simulink model "PVArrayGrid"  (R2024b)
settings: Solver=ode45  StartTime=0.0  StopTime=1.3  FixedStep=1  RelTol=1e-3
PreLoadFcn:
  | Ts_Power=1e-6;
  | Ts_Control=100e-6;
InitFcn:
  | Ts_Power=1e-6;
  | Ts_Control=100e-6;
undefined symbols (not defined in the file or in its folder): D1, Delta, DiscIntNeverNeededParam
libraries: spsSeriesRLCBranchLib x5, spsMeanLib x3, spsThreePhaseTransformerTwoWindingsLib x2, spsDistributedParametersLineLib x2, spsThreePhaseParallelRLCLoadLib x2, spsFourierLib x2, slpidlib x2, spsabctodq0Lib x2, spsVoltageMeasurementLib x2, spsThreePhaseSeriesRLCLoadLib x1, spsThreeLevelBridgeLib x1, spsThreePhaseSourceLib x1
(part 1 of 2)
settings Model: SimulationMode=accelerator  Creator=The MathWorks, Inc.  LastModifiedBy=shrot
settings SolverCC: AlgebraicLoopSolver=TrustRegion
settings DataIOCC: LimitDataPoints=on  SaveFormat=Array  SignalLogging=off  DSMLogging=off  ReturnWorkspaceOutputs=off
settings OptimizationCC: ExpressionDepthLimit=2147483647  EfficientMapNaN2IntZero=off  LifeSpan=inf
settings DebuggingCC: UnderspecifiedInitializationDetection=Classic  MergeDetectMultiDrivingBlocksExec=none  SolverPrmCheckMsg=warning  FcnCallInpInsideContextMsg=warning  UnconnectedInputMsg=warning  UnconnectedOutputMsg=warning  UnconnectedLineMsg=warning  StateNameClashWarn=warning  SubsystemReferenceDiagnosticForUnitTest=warning  SFUnexpectedBacktrackingDiag=warning  SFNoUnconditionalDefaultTransitionDiag=warning  SFExecutionAtInitializationDiag=none  ArithmeticOperatorsInVariantConditions=warning
settings HardwareCC: ProdBitPerPointer=32  ProdBitPerSizeT=32  ProdBitPerPtrDiffT=32  ProdLargestAtomicFloat=None  ProdIntDivRoundTo=Undefined  ProdEndianess=Unspecified  ProdWordSize=32  ProdHWDeviceType=32-bit Generic  TargetBitPerPointer=64  TargetBitPerSizeT=64  TargetBitPerPtrDiffT=64  TargetLongLongMode=on  TargetIntDivRoundTo=Zero  TargetEndianess=LittleEndian  TargetWordSize=64  TargetHWDeviceType=MATLAB Host  ProdEqTarget=off
settings ModelReferenceCC: EnableRefExpFcnMdlSchedulingChecks=on  PropagateSignalLabelsOutOfModel=off
settings SFSimCC: SimUseLocalCustomCode=off  CustomCodeUndefinedFunction=UseInterfaceOnly
settings RTWCC: GPUComputeCapability=3.5
settings CodeAppCC: MaxIdLength=128
settings GRTTargetCC: TargetLangStandard=C89/C90 (ANSI)  CombineOutputUpdateFcns=off  GRTInterface=on
settings ConfigComp: CovMetricSettings=dw  CovSaveCumulativeToWorkspaceVar=on  CovSaveSingleToWorkspaceVar=on  CovExternalEMLEnable=off  CovSFcnEnable=off
settings SimscapeCC: SimscapeNormalizeSystem=off

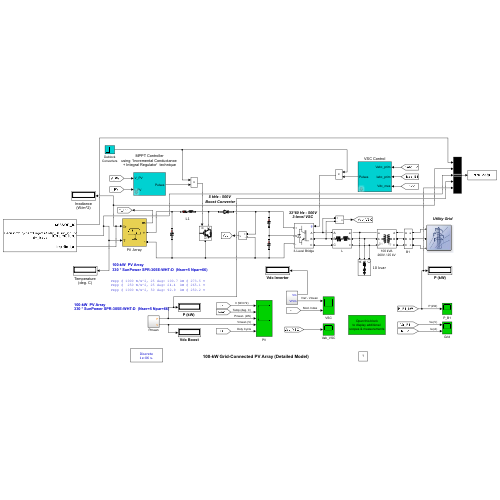
[thumbnail: Simulink's stored preview of the top-level diagram]
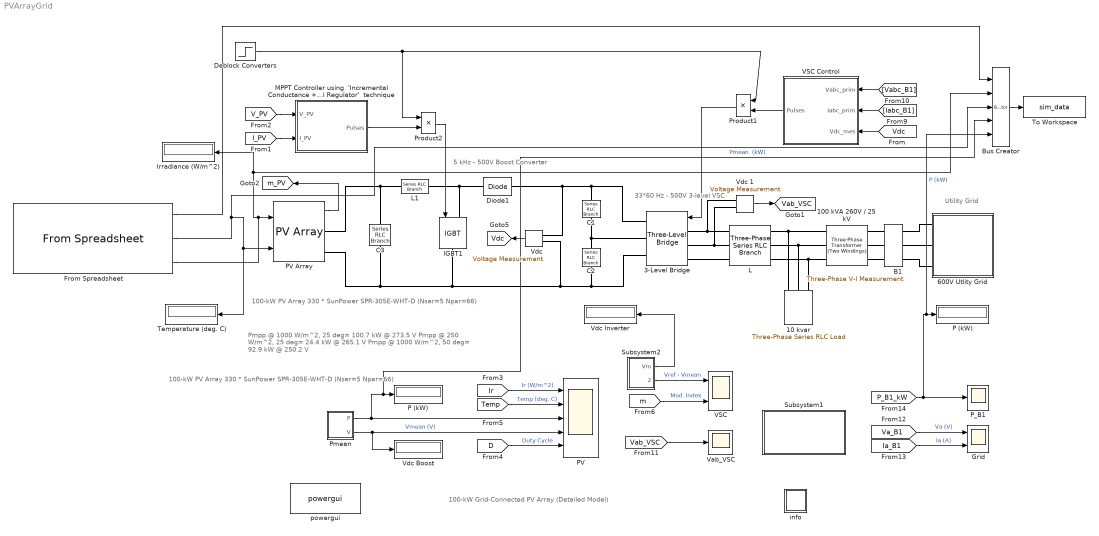
== system PVArrayGrid ==
  note: 5 kHz - 500V
      | Boost Converter
  note: 33*60 Hz - 500V
      | 3-level VSC
  note: 100-kW Grid-Connected PV Array (Detailed Model)
  note: Utility Grid
  note: Pmpp @ 1000 W/m^2, 25 deg= 100.7 kW @ 273.5 V
      | Pmpp @  250 W/m^2, 25 deg= 24.4  kW @ 265.1 V
      | Pmpp @ 1000 W/m^2, 50 deg= 92.9  kW @ 250.2 V
  note: 100-kW  PV Array
      | 330 * SunPower SPR-305E-WHT-D  (Nser=5 Npar=66)
  note: 100-kW  PV Array
      | 330 * SunPower SPR-305E-WHT-D  (Nser=5 Npar=66)
  10 kvar : spsThreePhaseSeriesRLCLoadLib/Three-Phase Series RLC Load  LConnTagsString=A|B|C  Configuration=Y (grounded)  NominalVoltage=240  Vabc=[1e3 1e3 1e3]  Vabcp=[1e3 1e3 1e3]  NominalFrequency=60  UnbalancedPower=off  ActivePower=10e3/100  InductivePower=0  CapacitivePower=10e3  Pabc=[10e3 9e3 11e3]  QLabc=[100 90 110]  QCabc=[100 90 110]  Pabcp=[10e3 9e3 11e3]  QLabcp=[100 90 110]  QCabcp=[100 90 110]  Measurements=None  LoadType=constant Z
  100 kVA 260V / 25 kV : spsThreePhaseTransformerTwoWindingsLib/Three-Phase Transformer (Two Windings)  Winding1Connection=Yg  Winding2Connection=Delta (D1)  CoreType=Three single-phase transformers  SetSaturation=off  Hysteresis=off  DataFile='hysteresis'  SetInitialFlux=off  Measurements=None  UNITS=pu  NominalPower=[100e3 , 60 ]  Winding1=[ 25e3 , 0.001 , 0.03 ]  Winding2=[ 260 , 0.001 , 0.03 ]  Rm=500  Lm=500  L0=0.5  Saturation=[ 0,0 ; 0.0024,1.2 ; 1.0,1.52 ]  InitialFluxes=[ 0.8 , -0.8 , 0.7 ]  BreakLoop=off  DiscreteSolver=Trapezoidal iterative  DataType=off  TransfoNumber=0
  3-Level Bridge : spsThreeLevelBridgeLib/Three-Level Bridge  Arms=3  SnubberResistance=1e6  SbubberCapacitance=inf  Device=IGBT / Diodes  Ron=0.2e-3  ForwardVoltages="[  0  0 ]"  Measurements=None
      settings: AttributesFormatString=\n
  600V Utlity Grid : Subsystem
      mask Display: image('$imagefile')
  B1 : spsThreePhaseVIMeasurementLib/Three-Phase V-I Measurement  VoltageMeasurement=phase-to-ground  SetLabelV=on  LabelV=Vabc_B1  Vpu=off  VpuLL=off  CurrentMeasurement=yes  SetLabelI=on  LabelI=Iabc_B1  Ipu=off  Pbase=100e6  Vbase=500e3  OutputType=Magnitude  PhasorSimulation=off  PSBequivalent=0
  Bus Creator : BusCreator  Inputs=5
  C1 : spsSeriesRLCBranchLib/Series RLC Branch  LConnTagsString=__new0  RConnTagsString=__new0  BranchType=C  Resistance=1.0  Inductance=1.0  SetiL0=off  InitialCurrent=0  Capacitance=12000e-06  Setx0=off  InitialVoltage=0  Measurements=None
  C2 : spsSeriesRLCBranchLib/Series RLC Branch  LConnTagsString=__new0  RConnTagsString=__new0  BranchType=C  Resistance=1.0  Inductance=1.0  SetiL0=off  InitialCurrent=0  Capacitance=12000e-06  Setx0=off  InitialVoltage=0  Measurements=None
  C3 : spsSeriesRLCBranchLib/Series RLC Branch  LConnTagsString=__new0  RConnTagsString=__new0  BranchType=C  Resistance=1.0  Inductance=1.0  SetiL0=off  InitialCurrent=0  Capacitance=100e-6  Setx0=off  InitialVoltage=0  Measurements=Branch voltage
  Deblock Converters : Step  Time=0.05  SampleTime=0
  Diode1 : spsDiodeLib/Diode  Ron=1e-4  Lon=0  Vf=0  IC=0  UseSnubber=off  Rs=inf  Cs=inf  Measurements=off
  From Spreadsheet : FromSpreadsheet  FileName=C:\Users\shrot\PycharmProjects\Solar_DT\sim_input.csv  SheetName=sim_input  TreatFirstColumnAs=Data  SampleTime=4
  Grid : Scope  NumInputPorts=2
  IGBT1 : spsIGBTLib/IGBT  Ron=0.001  Lon=0  Vf=0  Tf=0  Tt=0  IC=0  Rs=1e5  Cs=inf  Measurements=off
  Irradiance (W/m^2) : Display
      settings: Format=bank  Decimation=1000
  L : spsThreePhaseSeriesRLCBranchLib/Three-Phase Series RLC Branch  LConnTagsString=A|B|C  RConnTagsString=A|B|C  BranchType=RL  Resistance=500e-6*377/50/2  Inductance=500e-6/2  Capacitance=inf  Measurements=None
  L1 : spsSeriesRLCBranchLib/Series RLC Branch  LConnTagsString=__new0  RConnTagsString=__new0  BranchType=RL  Resistance=0.005  Inductance=5e-3  SetiL0=off  InitialCurrent=0  Capacitance=1e-6  Setx0=off  InitialVoltage=0  Measurements=None
  "MPPT Controller using  'Incremental Conductance + Integral Regulator'  technique " : Subsystem  mask(Boost Control - MPPT){fc=5000, T_MPPT=200e-6, Dinit=0.5}
      mask prompts: fc "PWM switching frequency (Hz)"; T_MPPT "Time window used by MPPT control (s)"; Dinit "Initial value of duty cycle"
  P (kW) : Display
      settings: Format=bank  Decimation=2000
  "P (kW) " : Display
      settings: Format=bank  Decimation=2000
  PV : Scope  NumInputPorts=5
  PV Array : spsPVArrayLib/PV Array  Npar=66  Nser=5  PlotType=array @ 1000 W/m2 & specified temperatures  S_vec="[ 1000  250 ]"  Temp_C_vec="[0 25 50  ]"  ModuleName=SunPower SPR-305E-WHT-D  PlotWhenSelected=off  Pm=305.226  Ncell=96  Voc=64.2  Isc=5.96  Vm=54.7  Im=5.58  beta_Voc_pc=-0.2727  alpha_Isc_pc=0.061745  beta_Voc=-0.17507  alpha_Isc=0.00368  IL=5.9657  I0=6.3076e-12  nI=0.94489  Rsh=393.2054  Rs=0.37428  RobustModel=off  RobustCellTemperature=25  BAL=on  Tc=1e-6  Tfilter=5e-5
  P_B1 : Scope
  Pmean : Subsystem
  Product1 : Product  RndMeth=Zero
  Product2 : Product  RndMeth=Zero
  Subsystem1 : Subsystem
      mask Display: disp('Open this block\nto display additional \nscopes & measurements')
  Subsystem2 : Subsystem
  Temperature (deg. C) : Display
      settings: Format=bank  Decimation=1000
  To Workspace : ToWorkspace  VariableName=sim_data  SampleTime=-1
      settings: MaxDataPoints=1
  VSC : Scope  NumInputPorts=2
  VSC Control : Subsystem  mask(VSC Main Controller){nom=[ 100e3  60 ], Vnom=[ 25e3 260 ], Vnom_dc=500, RLxfo=[0.002  0.06 ], RLchoke=[2e-3  250e-6  ], K_VDCreg=[7  800], K_Ireg=[0.3 20], Ts=Ts_Control}
      mask prompts: nom "Nominal power and frequency [ Pnom(VA)  Fnom(Hz) ]:"; Vnom "Nominal primary and secondary voltages (Vrms LL) [ Vnom_prim   Vnom_sec ]:"; Vnom_dc "Nominal DC bus voltage (V):"; RLxfo "Total transformer leakage impedance (pu/Pnom) [ Rxfo  Lxf ]"; RLchoke "Choke impedance [ R(ohm) L(H) ]"; K_VDCreg "VDC regultator gains [ Kp  Ki ]:"; K_Ireg "Current regulator gains [ Kp  Ki ]:"; Ts "Sample time"
      mask init:
      | Pnom=nom(1);
      | Fnom=nom(2);
      | Vnom_prim=Vnom(1);
      | Vnom_sec=Vnom(2);
      | Zbase=Vnom_sec^2/Pnom;
      | Rtot_pu=RLxfo(1) + RLchoke(1)/Zbase;
      | Ltot_pu=RLxfo(2) + RLchoke(2)/(Zbase/(2*pi*Fnom));
      | Kp_VDCreg=K_VDCreg(1);
      | Ki_VDCreg=K_VDCreg(2);
      | Kp_Ireg=K_Ireg(1);
      | Ki_Ireg=K_Ireg(2);
      | Vdc_ref=Vnom_dc;
      | % Used to determine initial value of Boost Control (MPPT)
      | assignin('base','Vdc_ref_Inv',Vdc_ref);
  Vab_VSC : Scope
  "Vdc " : spsVoltageMeasurementLib/Voltage Measurement  Tag=PoWeRsYsTeMmEaSuReMeNt  PhasorSimulation=off  OutputType=Magnitude  PSBequivalent=0
  Vdc 1 : spsVoltageMeasurementLib/Voltage Measurement  Tag=PoWeRsYsTeMmEaSuReMeNt  PhasorSimulation=off  OutputType=Magnitude  PSBequivalent=0
  Vdc Boost : Display
      settings: Format=bank  Decimation=2000
  Vdc Inverter : Display
      settings: Format=bank  Decimation=2000
  info : Subsystem
      settings: OpenFcn="showExample(\"simscapeelectricalsps/PVArrayGridExample\")"
      mask Display: disp('?')
  powergui : spspowerguiLib/powergui  Priority=1  SimulationMode=Discrete  SampleTime=Ts_Power  frequency=60  Iterations=50  frequencyindice=0  Pbase=100e6  ErrMax=1e-4  UnitsV=kV  UnitsW=MW  buscounter=0  FunctionMessages=off  echomessages=off  EnableUseOfTLC=off  CurrentSourceSwitches=off  DisableSnubberDevices=off  DisableRonSwitches=off  DisableVfSwitches=off  DisplayEquations=off  AutomaticDiscreteSolvers=off  SolverType=Tustin/Backward Euler (TBE)  Interpol=off  ExternalGateDelay=off  methode=off  Ts=0  x0status=blocks  SPID=off  SwTol=0  HookPort=off  NonlinearTolerance=1e-8  nMaxIteration=10  ContinueOnMaxIteration=off  RestoreLinks=warning  ResistiveCurrentMeasurement=off  Frange=[0:2:500]  Ylog=off  Xlog=on  ShowGrid=off  save=off  variable=ZData  structure=0  ZoomFFT=on  StartTime=0.0  cycles=1  DisplayStyle=1  fundamental=60  FreqAxis=off  MaxFrequency=1000  frequencyindicesteady=1  RmsSteady=1  display=off
  tag scope: Vab_VSC=global, Vdc=global, m_PV=global
  wires:
  "Vdc "/1 -> [Vdc]
  Product2/1 -> IGBT1/1
  "MPPT Controller using  'Incremental Conductance + Integral Regulator'  technique "/1(Pulses) -> Product2/2
  Deblock Converters/1 -> Product1/1, Product2/1
  [Vabc_B1] -> VSC Control/1(Vabc_prim)
  [Iabc_B1] -> VSC Control/2(Iabc_prim)
  [Vdc] -> VSC Control/3(Vdc_mes)
  VSC Control/1(Pulses) -> Product1/2
  Product1/1 -> 3-Level Bridge/1
  [I_PV] -> "MPPT Controller using  'Incremental Conductance + Integral Regulator'  technique "/2(I_PV)
  [V_PV] -> "MPPT Controller using  'Incremental Conductance + Integral Regulator'  technique "/1(V_PV)
  Pmean/1(P) -> Bus Creator/4, "P (kW) "/1, PV/3  "Pmean  (kW)"
  [m] -> VSC/2  "Mod. Index"
  Vdc 1/1 -> [Vab_VSC]
  [Vab_VSC] -> Vab_VSC/1
  [Ia_B1] -> Grid/2  "Ia (A)"
  [Va_B1] -> Grid/1  "Va (V)"
  [P_B1_kW] -> P_B1/1, Bus Creator/5, P (kW)/1  "P (kW)"
  Pmean/2(V) -> Vdc Boost/1, PV/4  "Vmean (V)"
  Subsystem2/2(VrVm) -> VSC/1  "Vref - Vmean"
  Subsystem2/1(Vm) -> Vdc Inverter/1
  PV Array/1 -> [m_PV]
  From Spreadsheet/2 -> Bus Creator/3, Temperature (deg. C)/1, PV Array/2
  [D] -> PV/5  "Duty Cycle"
  [Temp] -> PV/2  "Temp (deg. C)"
  [Ir] -> PV/1  "Ir (W/m^2)"
  Bus Creator/1 -> To Workspace/1
  From Spreadsheet/3 -> PV Array/1, Bus Creator/2, Irradiance (W/m^2)/1
  From Spreadsheet/1 -> Bus Creator/1
  connections:
  3-Level Bridge/RConn1 -- Diode1/RConn1 -- "Vdc "/LConn1 -- C1/LConn1
  L1/RConn1 -- Diode1/LConn1 -- IGBT1/LConn1
  3-Level Bridge/RConn3 -- C2/RConn1 -- "Vdc "/LConn2 -- IGBT1/RConn1 -- PV Array/RConn2 -- C3/RConn1
  3-Level Bridge/LConn1 -- L/LConn1 -- Vdc 1/LConn1
  3-Level Bridge/LConn2 -- L/LConn2 -- Vdc 1/LConn2
  3-Level Bridge/LConn3 -- L/LConn3
  L/RConn1 -- 100 kVA 260V / 25 kV/RConn1 -- 10 kvar/LConn1
  L/RConn2 -- 100 kVA 260V / 25 kV/RConn2 -- 10 kvar/LConn2
  L/RConn3 -- 100 kVA 260V / 25 kV/RConn3 -- 10 kvar/LConn3
  B1/LConn1 -- 100 kVA 260V / 25 kV/LConn1
  B1/LConn2 -- 100 kVA 260V / 25 kV/LConn2
  B1/LConn3 -- 100 kVA 260V / 25 kV/LConn3
  C2/LConn1 -- C1/RConn1 -- 3-Level Bridge/RConn2
  C3/LConn1 -- PV Array/RConn1 -- L1/LConn1
  B1/RConn2 -- 600V Utlity Grid/LConn2
  B1/RConn1 -- 600V Utlity Grid/LConn1
  B1/RConn3 -- 600V Utlity Grid/LConn3

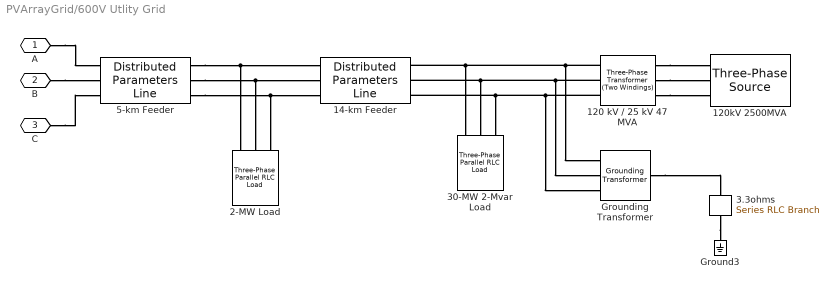
== system PVArrayGrid/600V Utlity Grid ==
  120 kV / 25 kV 47 MVA : spsThreePhaseTransformerTwoWindingsLib/Three-Phase Transformer (Two Windings)  Winding1Connection=Yg  Winding2Connection=Delta (D1)  CoreType=Three single-phase transformers  SetSaturation=off  Hysteresis=off  DataFile='basic_model'  SetInitialFlux=off  Measurements=None  UNITS=pu  NominalPower=[47e6 60 ]  Winding1="[ 120e3  0.08/30   0.08 ]"  Winding2="[ 25e3  0.08/30  0.08]"  Rm=500  Lm=500  L0=0.5  Saturation="[ 0,0  ;  0.005,1.2  ;  1.0,1.4 ]"  InitialFluxes=[ 0.8 , -0.8 , 0.7 ]  BreakLoop=off  DiscreteSolver=Trapezoidal iterative  DataType=off  TransfoNumber=0
  120kV 2500MVA : spsThreePhaseSourceLib/Three-Phase Source  InternalConnection=Yg  VoltagePhases=off  Voltage=120e3  PhaseAngle=0  Voltage_phases=[25e3 25e3 25e3]/sqrt(3)  PhaseAngles_phases=[0 -120 +120]  Frequency=60  NonIdealSource=on  SpecifyImpedance=on  Resistance=0.8929  Inductance=16.58e-3  ShortCircuitLevel=2500e6  BaseVoltage=120e3  XRratio=7  BusType=swing  Pref=0  Qref=0  Prefabc=[10e3, 10e3, 10e3]  Qrefabc=[0, 0, 0]  Qmin=-inf  Qmax=inf
  14-km Feeder : spsDistributedParametersLineLib/Distributed Parameters Line  Phases=3  Length=14  Frequency=60  Resistance=[0.1153 0.413]  Inductance=[1.05e-3 3.32e-3]  Capacitance=[11.33e-009 5.01e-009]  x1=[-5.8e-05 1.09765853041463e-09 0 0;-5.7e-05 1.09777450341744e-09 0 0;-5.6e-05 1.09789032040201e-09 0 0;-5.5e-05 1.09800598135188e-09 0 0;-5.4e-05 1.09812148625062e-09 0 0;-5.3e-05 1.0982368350818e-09 0 0;-5.2e-05 1.09835202782904e-09 0 0;-5.1e-05 1.09846706447595e-09 0 0;-5e-05 1.0985819450062e-09 0 0;-4.9e-05 1.09869666940346e-09 -3790.73535189818 -24061.4134200269;-4.8e-05 1.09881123765141e-09 -3781.66414358279 -24062.8407837213;-4.7e-05 1.09892564973379e-09 -3772.59239780858 -24064.2647275494;-4.6e-05 1.09903990563432e-09 -3763.52011586486 -24065.6852513088;-4.5e-05 1.09915400533677e-09 -3754.447299041 -24067.1023547976;-4.4e-05 1.09926794882492e-09 -3745.37394862644 -24068.5160378144;-4.3e-05 1.09938173608258e-09 -3736.30006591072 -24069.9263001584;-4.2e-05 1.09949536709358e-09 -3727.22565218343 -24071.333141629;-4.1e-05 1.09960884184177e-09 -3718.15070873426 -24072.7365620263;-4e-05 1.09972216031101e-09 -3709.07523685295 -24074.1365611509;-3.9e-05 1.09983532248522e-09 -3699.99923782933 -24075.5331388038;-3.8e-05 1.09994832834829e-09 -3690.9227129533 -24076.9262947866;-3.7e-05 1.10006117788418e-09 -3681.84566351484 -24078.3160289011;-3.6e-05 1.10017387107684e-09 -3672.768090804 -24079.70234095;-3.5e-05 1.10028640791025e-09 -3663.6899961109 -24081.0852307361;-3.4e-05 1.10039878836843e-09 -3654.61138072575 -24082.464698063;-3.3e-05 1.10051101243541e-09 -3645.53224593882 -24083.8407427345;-3.2e-05 1.10062308009522e-09 -3636.45259304045 -24085.2133645552;-3.1e-05 1.10073499133195e-09 -3627.37242332107 -24086.5825633299;-3e-05 1.10084674612968e-09 -3618.29173807118 -24087.9483388641;-2.9e-05 1.10095834447255e-09 -3609.21053858133 -24089.3106909636;-2.8e-05 1.10106978634468e-09 -3600.12882614218 -24090.6696194348;-2.7e-05 1.10118107173024e-09 -3591.04660204443 -24092.0251240846;-2.6e-05 1.10129220061341e-09 -3581.96386757887 -24093.3772047204;-2.5e-05 1.10140317297839e-09 -3572.88062403636 -24094.7258611499;-2.4e-05 1.10151398880943e-09 -3563.79687270783 -24096.0710931815;-2.3e-05 1.10162464809076e-09 -3554.71261488429 -24097.412900624;-2.2e-05 1.10173515080665e-09 -3545.62785185682 -24098.7512832868;-2.1e-05 1.10184549694142e-09 -3536.54258491655 -24100.0862409795;-2e-05 1.10195568647936e-09 -3527.4568153547 -24101.4177735126;-1.9e-05 1.10206571940483e-09 -3518.37054446258 -24102.7458806966;-1.8e-05 1.10217559570218e-09 -3509.28377353153 -24104.0705623429;-1.7e-05 1.1022853153558e-09 -3500.196503853 -24105.3918182633;-1.6e-05 1.10239487835009e-09 -3491.10873671849 -24106.7096482699;-1.5e-05 1.10250428466948e-09 -3482.02047341956 -24108.0240521754;-1.4e-05 1.10261353429843e-09 -3472.93171524788 -24109.335029793;-1.3e-05 1.1027226272214e-09 -3463.84246349514 -24110.6425809365;-1.2e-05 1.1028315634229e-09 -3454.75271945314 -24111.9467054199;-1.1e-05 1.10294034288744e-09 -3445.66248441373 -24113.247403058;-1e-05 1.10304896559955e-09 -3436.57175966884 -24114.5446736659;-9e-06 1.10315743154381e-09 -3427.48054651046 -24115.8385170591;-8e-06 1.10326574070479e-09 -3418.38884623065 -24117.1289330539;-7e-06 1.10337389306711e-09 -3409.29666012156 -24118.4159214668;-6e-06 1.10348188861539e-09 -3400.20398947537 -24119.6994821149;-5e-06 1.10358972733429e-09 -3391.11083558437 -24120.9796148158;-4e-06 1.10369740920847e-09 -3382.01719974089 -24122.2563193876;-3e-06 1.10380493422264e-09 -3372.92308323734 -24123.5295956488;-2e-06 1.10391230236151e-09 -3363.8284873662 -24124.7994434184;-1e-06 1.10401951360982e-09 -3354.73341342002 -24126.0658625161]  x2=[-5.8e-05 1.13481958980174e-09 0 0;-5.7e-05 1.13493792425514e-09 0 0;-5.6e-05 1.13505609740854e-09 0 0;-5.5e-05 1.13517410924515e-09 0 0;-5.4e-05 1.13529195974821e-09 0 0;-5.3e-05 1.13540964890097e-09 0 0;-5.2e-05 1.13552717668669e-09 0 0;-5.1e-05 1.13564454308867e-09 0 0;-5e-05 1.13576174809024e-09 0 0;-4.9e-05 1.13587879167473e-09 -3379.39242591167 -24244.051273217;-4.8e-05 1.13599567382552e-09 -3370.25239397986 -24245.3235513069;-4.7e-05 1.13611239452599e-09 -3361.11188306003 -24246.5923835956;-4.6e-05 1.13622895375954e-09 -3351.97089445124 -24247.8577699028;-4.5e-05 1.13634535150963e-09 -3342.82942945264 -24249.1197100486;-4.4e-05 1.13646158775969e-09 -3333.68748936342 -24250.3782038537;-4.3e-05 1.13657766249322e-09 -3324.54507548286 -24251.6332511393;-4.2e-05 1.13669357569372e-09 -3315.4021891103 -24252.8848517269;-4.1e-05 1.13680932734471e-09 -3306.25883154515 -24254.1330054387;-4e-05 1.13692491742974e-09 -3297.11500408689 -24255.3777120973;-3.9e-05 1.13704034593239e-09 -3287.97070803506 -24256.6189715258;-3.8e-05 1.13715561283624e-09 -3278.82594468926 -24257.8567835478;-3.7e-05 1.13727071812492e-09 -3269.68071534916 -24259.0911479873;-3.6e-05 1.13738566178207e-09 -3260.53502131452 -24260.322064669;-3.5e-05 1.13750044379135e-09 -3251.38886388514 -24261.5495334178;-3.4e-05 1.13761506413645e-09 -3242.24224436089 -24262.7735540594;-3.3e-05 1.13772952280108e-09 -3233.09516404171 -24263.9941264198;-3.2e-05 1.13784381976897e-09 -3223.9476242276 -24265.2112503254;-3.1e-05 1.13795795502387e-09 -3214.79962621864 -24266.4249256034;-3e-05 1.13807192854958e-09 -3205.65117131495 -24267.6351520813;-2.9e-05 1.13818574032988e-09 -3196.50226081674 -24268.8419295869;-2.8e-05 1.1382993903486e-09 -3187.35289602427 -24270.0452579489;-2.7e-05 1.1384128785896e-09 -3178.20307823788 -24271.2451369962;-2.6e-05 1.13852620503673e-09 -3169.05280875794 -24272.4415665583;-2.5e-05 1.1386393696739e-09 -3159.90208888493 -24273.6345464651;-2.4e-05 1.13875237248503e-09 -3150.75091991935 -24274.8240765471;-2.3e-05 1.13886521345404e-09 -3141.59930316181 -24276.0101566352;-2.2e-05 1.13897789256491e-09 -3132.44723991294 -24277.1927865609;-2.1e-05 1.13909040980162e-09 -3123.29473147346 -24278.3719661561;-2e-05 1.13920276514818e-09 -3114.14177914414 -24279.5476952531;-1.9e-05 1.13931495858862e-09 -3104.98838422583 -24280.719973685;-1.8e-05 1.13942699010699e-09 -3095.83454801942 -24281.888801285;-1.7e-05 1.13953885968738e-09 -3086.68027182588 -24283.0541778872;-1.6e-05 1.13965056731389e-09 -3077.52555694623 -24284.2161033257;-1.5e-05 1.13976211297063e-09 -3068.37040468157 -24285.3745774356;-1.4e-05 1.13987349664176e-09 -3059.21481633304 -24286.5296000522;-1.3e-05 1.13998471831144e-09 -3050.05879320186 -24287.6811710113;-1.2e-05 1.14009577796387e-09 -3040.90233658931 -24288.8292901492;-1.1e-05 1.14020667558326e-09 -3031.74544779671 -24289.9739573028;-1e-05 1.14031741115386e-09 -3022.58812812548 -24291.1151723093;-9e-06 1.14042798465992e-09 -3013.43037887706 -24292.2529350067;-8e-06 1.14053839608573e-09 -3004.27220135299 -24293.3872452332;-7e-06 1.1406486454156e-09 -2995.11359685483 -24294.5181028276;-6e-06 1.14075873263386e-09 -2985.95456668423 -24295.6455076291;-5e-06 1.14086865772486e-09 -2976.7951121429 -24296.7694594776;-4e-06 1.14097842067298e-09 -2967.6352345326 -24297.8899582133;-3e-06 1.14108802146262e-09 -2958.47493515514 -24299.0070036769;-2e-06 1.14119746007821e-09 -2949.31421531242 -24300.1205957098;-1e-06 1.14130673650419e-09 -2940.15307630637 -24301.2307341535]  x3=[-5.8e-05 1.57399423716255e-12 0 0;-5.7e-05 1.57518382731474e-12 0 0;-5.6e-05 1.57637319359817e-12 0 0;-5.5e-05 1.57756233584382e-12 0 0;-5.4e-05 1.57875125388268e-12 0 0;-5.3e-05 1.57993994754577e-12 0 0;-5.2e-05 1.58112841666416e-12 0 0;-5.1e-05 1.58231666106895e-12 0 0;-5e-05 1.58350468059125e-12 0 0;-4.9e-05 1.58469247506221e-12 -23.5442847382529 -155.681477773836;-4.8e-05 1.58588004431304e-12 -23.4855925321342 -155.690342696957;-4.7e-05 1.58706738817494e-12 -23.4268969881891 -155.699185493008;-4.6e-05 1.58825450647917e-12 -23.3681981147594 -155.708006160732;-4.5e-05 1.58944139905702e-12 -23.3094959201876 -155.716804698876;-4.4e-05 1.5906280657398e-12 -23.2507904128166 -155.72558110619;-4.3e-05 1.59181450635885e-12 -23.1920816009898 -155.734335381425;-4.2e-05 1.59300072074557e-12 -23.1333694930509 -155.743067523339;-4.1e-05 1.59418670873135e-12 -23.0746540973444 -155.751777530689;-4e-05 1.59537247014765e-12 -23.0159354222148 -155.760465402238;-3.9e-05 1.59655800482594e-12 -22.9572134760076 -155.769131136751;-3.8e-05 1.59774331259774e-12 -22.8984882670684 -155.777774732996;-3.7e-05 1.59892839329458e-12 -22.8397598037432 -155.786396189746;-3.6e-05 1.60011324674803e-12 -22.7810280943789 -155.794995505775;-3.5e-05 1.60129787278971e-12 -22.7222931473224 -155.80357267986;-3.4e-05 1.60248227125124e-12 -22.6635549709213 -155.812127710783;-3.3e-05 1.60366644196431e-12 -22.6048135735236 -155.820660597327;-3.2e-05 1.60485038476061e-12 -22.5460689634778 -155.829171338281;-3.1e-05 1.60603409947188e-12 -22.4873211491327 -155.837659932434;-3e-05 1.60721758592989e-12 -22.4285701388378 -155.84612637858;-2.9e-05 1.60840084396644e-12 -22.3698159409429 -155.854570675516;-2.8e-05 1.60958387341335e-12 -22.3110585637983 -155.862992822042;-2.7e-05 1.61076667410251e-12 -22.2522980157547 -155.871392816961;-2.6e-05 1.61194924586579e-12 -22.1935343051632 -155.879770659078;-2.5e-05 1.61313158853514e-12 -22.1347674403756 -155.888126347204;-2.4e-05 1.61431370194251e-12 -22.0759974297439 -155.89645988015;-2.3e-05 1.6154955859199e-12 -22.0172242816206 -155.904771256732;-2.2e-05 1.61667724029935e-12 -21.9584480043588 -155.91306047577;-2.1e-05 1.6178586649129e-12 -21.8996686063117 -155.921327536085;-2e-05 1.61903985959265e-12 -21.8408860958334 -155.929572436501;-1.9e-05 1.62022082417074e-12 -21.782100481278 -155.937795175848;-1.8e-05 1.62140155847931e-12 -21.7233117710004 -155.945995752956;-1.7e-05 1.62258206235056e-12 -21.6645199733557 -155.954174166661;-1.6e-05 1.62376233561671e-12 -21.6057250966996 -155.9623304158;-1.5e-05 1.62494237811002e-12 -21.5469271493881 -155.970464499213;-1.4e-05 1.62612218966278e-12 -21.4881261397777 -155.978576415744;-1.3e-05 1.62730177010731e-12 -21.4293220762254 -155.986666164242;-1.2e-05 1.62848111927597e-12 -21.3705149670885 -155.994733743555;-1.1e-05 1.62966023700114e-12 -21.3117048207248 -156.002779152538;-1e-05 1.63083912311525e-12 -21.2528916454926 -156.010802390047;-9e-06 1.63201777745075e-12 -21.1940754497505 -156.018803454941;-8e-06 1.63319619984013e-12 -21.1352562418576 -156.026782346084;-7e-06 1.63437439011591e-12 -21.0764340301734 -156.034739062341;-6e-06 1.63555234811063e-12 -21.017608823058 -156.042673602583;-5e-06 1.63673007365689e-12 -20.9587806288716 -156.05058596568;-4e-06 1.6379075665873e-12 -20.899949455975 -156.058476150509;-3e-06 1.63908482673453e-12 -20.8411153127295 -156.066344155948;-2e-06 1.64026185393124e-12 -20.7822782074968 -156.074189980879;-1e-06 1.64143864801016e-12 -20.7234381486388 -156.082013624187]  x4=[-5.8e-05 1.05853260132924e-12 0 0;-5.7e-05 1.0580479194887e-12 0 0;-5.6e-05 1.05756308727595e-12 0 0;-5.5e-05 1.0570781047599e-12 0 0;-5.4e-05 1.05659297200948e-12 0 0;-5.3e-05 1.05610768909363e-12 0 0;-5.2e-05 1.05562225608133e-12 0 0;-5.1e-05 1.05513667304156e-12 0 0;-5e-05 1.05465094004334e-12 0 0;-4.9e-05 1.0541650571557e-12 -1.35581366009422 -2.15298522698177;-4.8e-05 1.05367902444769e-12 -1.35500190745908 -2.15349620368416;-4.7e-05 1.0531928419884e-12 -1.35418996224795 -2.15400687432671;-4.6e-05 1.05270650984692e-12 -1.35337782457623 -2.15451723883685;-4.5e-05 1.05222002809236e-12 -1.35256549455934 -2.15502729714204;-4.4e-05 1.05173339679387e-12 -1.35175297231272 -2.15553704916979;-4.3e-05 1.05124661602062e-12 -1.35094025795186 -2.15604649484765;-4.2e-05 1.05075968584177e-12 -1.35012735159227 -2.15655563410322;-4.1e-05 1.05027260632654e-12 -1.34931425334946 -2.15706446686414;-4e-05 1.04978537754414e-12 -1.34850096333901 -2.1575729930581;-3.9e-05 1.04929799956384e-12 -1.3476874816765 -2.15808121261281;-3.8e-05 1.04881047245488e-12 -1.34687380847754 -2.15858912545605;-3.7e-05 1.04832279628657e-12 -1.34605994385778 -2.15909673151564;-3.6e-05 1.04783497112821e-12 -1.34524588793287 -2.15960403071944;-3.5e-05 1.04734699704913e-12 -1.34443164081853 -2.16011102299533;-3.4e-05 1.04685887411869e-12 -1.34361720263047 -2.16061770827128;-3.3e-05 1.04637060240625e-12 -1.34280257348443 -2.16112408647527;-3.2e-05 1.04588218198121e-12 -1.34198775349621 -2.16163015753532;-3.1e-05 1.04539361291299e-12 -1.3411727427816 -2.16213592137952;-3e-05 1.04490489527103e-12 -1.34035754145642 -2.16264137793599;-2.9e-05 1.04441602912477e-12 -1.33954214963655 -2.16314652713289;-2.8e-05 1.04392701454371e-12 -1.33872656743787 -2.16365136889843;-2.7e-05 1.04343785159734e-12 -1.33791079497629 -2.16415590316085;-2.6e-05 1.04294854035517e-12 -1.33709483236774 -2.16466012984845;-2.5e-05 1.04245908088676e-12 -1.3362786797282 -2.16516404888958;-2.4e-05 1.04196947326167e-12 -1.33546233717366 -2.1656676602126;-2.3e-05 1.04147971754947e-12 -1.33464580482013 -2.16617096374595;-2.2e-05 1.04098981381978e-12 -1.33382908278368 -2.1666739594181;-2.1e-05 1.04049976214223e-12 -1.33301217118036 -2.16717664715756;-2e-05 1.04000956258645e-12 -1.33219507012628 -2.16767902689289;-1.9e-05 1.03951921522212e-12 -1.33137777973758 -2.16818109855268;-1.8e-05 1.03902872011892e-12 -1.3305603001304 -2.16868286206559;-1.7e-05 1.03853807734658e-12 -1.32974263142093 -2.1691843173603;-1.6e-05 1.03804728697481e-12 -1.32892477372537 -2.16968546436553;-1.5e-05 1.03755634907337e-12 -1.32810672715997 -2.17018630301008;-1.4e-05 1.03706526371203e-12 -1.32728849184098 -2.17068683322275;-1.3e-05 1.03657403096059e-12 -1.3264700678847 -2.17118705493242;-1.2e-05 1.03608265088887e-12 -1.32565145540744 -2.17168696806798;-1.1e-05 1.03559112356669e-12 -1.32483265452554 -2.17218657255839;-1e-05 1.03509944906392e-12 -1.32401366535538 -2.17268586833265;-9e-06 1.03460762745043e-12 -1.32319448801334 -2.17318485531979;-8e-06 1.03411565879613e-12 -1.32237512261586 -2.1736835334489;-7e-06 1.03362354317093e-12 -1.32155556927938 -2.17418190264909;-6e-06 1.03313128064477e-12 -1.32073582812039 -2.17467996284956;-5e-06 1.03263887128761e-12 -1.31991589925538 -2.1751777139795;-4e-06 1.03214631516945e-12 -1.31909578280088 -2.17567515596818;-3e-06 1.03165361236027e-12 -1.31827547887345 -2.17617228874489;-2e-06 1.0311607629301e-12 -1.31745498758968 -2.176669112239;-1e-06 1.030667766949e-12 -1.31663430906618 -2.17716562637988]  x5=5.70973484498186e-05  V1=[0 0 0 2.868e-09 2.436e+04 2.436e+04;0 0 0 377 377 377;1.571 1.571 1.571 -0.5389 -0.156 -1.727]  V2=[0 0 0 2.996e-09 2.448e+04 2.448e+04;0 0 0 377 377 377;1.571 1.571 1.571 -0.5232 -0.1382 -1.709]  I1=[0 0 0 1.022e-11 157.5 157.5;0 0 0 377 377 377;1.571 1.571 1.571 -1.198 -0.1498 -1.721]  I2=[0 0 0 6.231e-12 2.544 2.544;0 0 0 377 377 377;1.571 1.571 1.571 1.184 -0.5617 -2.133]  nHarmo=2  Measurements=None  Decoupling=off  VsMag0=0  VrMag0=0  VsAngle0=0  VrAngle0=0  IsMag0=0  IrMag0=0  IsAngle0=0  IrAngle0=0
  2-MW Load : spsThreePhaseParallelRLCLoadLib/Three-Phase Parallel RLC Load  LConnTagsString=A|B|C  Configuration=Y (grounded)  NominalVoltage=25e3  Vabc=[1e3 1e3 1e3]  Vabcp=[1e3 1e3 1e3]  NominalFrequency=60  UnbalancedPower=off  ActivePower=2e6  InductivePower=0  CapacitivePower=0  Pabc=[10e3 9e3 11e3]  QLabc=[100 90 110]  QCabc=[100 90 110]  Pabcp=[10e3 9e3 11e3]  QLabcp=[100 90 110]  QCabcp=[100 90 110]  Measurements=None  LoadType=constant Z
  "3.3ohms " : spsSeriesRLCBranchLib/Series RLC Branch  LConnTagsString=__new0  RConnTagsString=__new0  BranchType=R  Resistance=3.3  Inductance=[]  SetiL0=off  InitialCurrent=0  Capacitance=[]  Setx0=off  InitialVoltage=0  Measurements=None
  30-MW 2-Mvar Load : spsThreePhaseParallelRLCLoadLib/Three-Phase Parallel RLC Load  LConnTagsString=A|B|C  Configuration=Y (grounded)  NominalVoltage=25e3  Vabc=[1e3 1e3 1e3]  Vabcp=[1e3 1e3 1e3]  NominalFrequency=60  UnbalancedPower=off  ActivePower=30e6  InductivePower=2e6  CapacitivePower=0  Pabc=[10e3 9e3 11e3]  QLabc=[100 90 110]  QCabc=[100 90 110]  Pabcp=[10e3 9e3 11e3]  QLabcp=[100 90 110]  QCabcp=[100 90 110]  Measurements=None  LoadType=constant Z
  5-km Feeder : spsDistributedParametersLineLib/Distributed Parameters Line  Phases=3  Length=5  Frequency=60  Resistance=[0.1153 0.413]  Inductance=[1.05e-3 3.32e-3]  Capacitance=[11.33e-009 5.01e-009]  x1=[-2.1e-05 1.08380017743144e-09 -3537.17773129479 -24101.4118174708;-2e-05 1.08390345674986e-09 -3528.09146195726 -24102.7435893542;-1.9e-05 1.08400658202142e-09 -3519.00469119925 -24104.0719357001;-1.8e-05 1.08410955323147e-09 -3509.9174203122 -24105.3968563199;-1.7e-05 1.08421237036538e-09 -3500.8296505876 -24106.7183510252;-1.6e-05 1.08431503340852e-09 -3491.74138331704 -24108.0364196282;-1.5e-05 1.08441754234632e-09 -3482.65261979215 -24109.3510619416;-1.4e-05 1.08451989716421e-09 -3473.56336130466 -24110.6622777785;-1.3e-05 1.08462209784762e-09 -3464.47360914634 -24111.9700669526;-1.2e-05 1.08472414438205e-09 -3455.38336460907 -24113.274429278;-1.1e-05 1.08482603675299e-09 -3446.29262898475 -24114.5753645693;-1e-05 1.08492777494596e-09 -3437.2014035654 -24115.8728726417;-9e-06 1.08502935894649e-09 -3428.10968964307 -24117.1669533107;-8e-06 1.08513078874015e-09 -3419.0174885099 -24118.4576063925;-7e-06 1.08523206431253e-09 -3409.9248014581 -24119.7448317035;-6e-06 1.08533318564922e-09 -3400.83162977993 -24121.0286290609;-5e-06 1.08543415273587e-09 -3391.73797476775 -24122.3089982822;-4e-06 1.08553496555812e-09 -3382.64383771395 -24123.5859391854;-3e-06 1.08563562410164e-09 -3373.54921991103 -24124.8594515891;-2e-06 1.08573612835212e-09 -3364.45412265153 -24126.1295353122;-1e-06 1.08583647829529e-09 -3355.35854722807 -24127.3961901742]  x2=[-2.1e-05 1.10184549694142e-09 -3536.54258491655 -24100.0862409795;-2e-05 1.10195568647936e-09 -3527.4568153547 -24101.4177735126;-1.9e-05 1.10206571940483e-09 -3518.37054446258 -24102.7458806966;-1.8e-05 1.10217559570218e-09 -3509.28377353153 -24104.0705623429;-1.7e-05 1.1022853153558e-09 -3500.196503853 -24105.3918182633;-1.6e-05 1.10239487835009e-09 -3491.10873671849 -24106.7096482699;-1.5e-05 1.10250428466948e-09 -3482.02047341956 -24108.0240521754;-1.4e-05 1.10261353429843e-09 -3472.93171524788 -24109.335029793;-1.3e-05 1.1027226272214e-09 -3463.84246349514 -24110.6425809365;-1.2e-05 1.1028315634229e-09 -3454.75271945314 -24111.9467054199;-1.1e-05 1.10294034288744e-09 -3445.66248441373 -24113.247403058;-1e-05 1.10304896559955e-09 -3436.57175966884 -24114.5446736659;-9e-06 1.10315743154381e-09 -3427.48054651046 -24115.8385170591;-8e-06 1.10326574070479e-09 -3418.38884623065 -24117.1289330539;-7e-06 1.10337389306711e-09 -3409.29666012156 -24118.4159214668;-6e-06 1.10348188861539e-09 -3400.20398947537 -24119.6994821149;-5e-06 1.10358972733429e-09 -3391.11083558437 -24120.9796148158;-4e-06 1.10369740920847e-09 -3382.01719974089 -24122.2563193876;-3e-06 1.10380493422264e-09 -3372.92308323734 -24123.5295956488;-2e-06 1.10391230236151e-09 -3363.8284873662 -24124.7994434184;-1e-06 1.10401951360982e-09 -3354.73341342002 -24126.0658625161]  x3=[-2.1e-05 -9.48542028854319e-13 -11.1569792961328 -79.1361755515074;-2e-05 -9.4696699220072e-13 -11.1271448686821 -79.1403760100032;-1.9e-05 -9.45391820961993e-13 -11.0973088598161 -79.1445652208866;-1.8e-05 -9.43816515362004e-13 -11.0674712737749 -79.1487431835623;-1.7e-05 -9.4224107562464e-13 -11.0376321147993 -79.1529098974364;-1.6e-05 -9.40665501973805e-13 -11.00779138713 -79.1570653619168;-1.5e-05 -9.39089794633424e-13 -10.9779490950081 -79.1612095764128;-1.4e-05 -9.3751395382744e-13 -10.9481052426747 -79.1653425403355;-1.3e-05 -9.35937979779815e-13 -10.9182598343715 -79.1694642530975;-1.2e-05 -9.3436187271453e-13 -10.88841287434 -79.173574714113;-1.1e-05 -9.32785632855585e-13 -10.8585643668222 -79.1776739227979;-1e-05 -9.31209260426999e-13 -10.8287143160602 -79.1817618785695;-9e-06 -9.29632755652809e-13 -10.7988627262965 -79.1858385808469;-8e-06 -9.28056118757073e-13 -10.7690096017735 -79.1899040290506;-7e-06 -9.26479349963865e-13 -10.7391549467341 -79.1939582226029;-6e-06 -9.24902449497279e-13 -10.7092987654213 -79.1980011609275;-5e-06 -9.23325417581428e-13 -10.6794410620783 -79.20203284345;-4e-06 -9.21748254440443e-13 -10.6495818409485 -79.2060532695972;-3e-06 -9.20170960298475e-13 -10.6197211062757 -79.2100624387979;-2e-06 -9.18593535379693e-13 -10.5898588623036 -79.2140603504821;-1e-06 -9.17015979908282e-13 -10.5599951132765 -79.2180470040818]  x4=[-2.1e-05 2.26150729240339e-12 -12.5606324025971 -78.9000787577133;-2e-05 2.25992805505108e-12 -12.5308868817935 -78.9048083977284;-1.9e-05 2.25834849651259e-12 -12.5011395800715 -78.9095268236105;-1.8e-05 2.25676861701241e-12 -12.4713905016587 -78.9142340346891;-1.7e-05 2.25518841677508e-12 -12.4416396507832 -78.918930030295;-1.6e-05 2.25360789602518e-12 -12.4118870316732 -78.923614809761;-1.5e-05 2.25202705498734e-12 -12.3821326485572 -78.9282883724212;-1.4e-05 2.25044589388624e-12 -12.3523765056641 -78.9329507176113;-1.3e-05 2.24886441294658e-12 -12.3226186072228 -78.9376018446688;-1.2e-05 2.24728261239313e-12 -12.2928589574626 -78.9422417529327;-1.1e-05 2.24570049245071e-12 -12.2630975606129 -78.9468704417435;-1e-05 2.24411805334417e-12 -12.2333344209036 -78.9514879104433;-9e-06 2.2425352952984e-12 -12.2035695425647 -78.9560941583759;-8e-06 2.24095221853836e-12 -12.1738029298264 -78.9606891848867;-7e-06 2.23936882328902e-12 -12.1440345869192 -78.9652729893226;-6e-06 2.23778510977544e-12 -12.1142645180738 -78.9698455710322;-5e-06 2.23620107822268e-12 -12.0844927275213 -78.9744069293655;-4e-06 2.23461672885589e-12 -12.0547192194928 -78.9789570636744;-3e-06 2.23303206190021e-12 -12.0249439982199 -78.9834959733121;-2e-06 2.23144707758089e-12 -11.9951670679343 -78.9880236576335;-1e-06 2.22986177612316e-12 -11.965388432868 -78.9925401159953]  x5=2.03919101606495e-05  V1=[0 0 0 2.827e-09 2.436e+04 2.436e+04;0 0 0 377 377 377;1.571 1.571 1.571 -0.5179 -0.1443 -1.715]  V2=[0 0 0 2.868e-09 2.436e+04 2.436e+04;0 0 0 377 377 377;1.571 1.571 1.571 -0.5251 -0.1443 -1.715]  I1=[0 0 0 7.018e-12 79.92 79.92;0 0 0 377 377 377;1.571 1.571 1.571 -1.622 -0.1386 -1.709]  I2=[0 0 0 7.946e-12 79.89 79.89;0 0 0 377 377 377;1.571 1.571 1.571 0.3547 -0.1565 -1.727]  nHarmo=2  Measurements=None  Decoupling=off  VsMag0=0  VrMag0=0  VsAngle0=0  VrAngle0=0  IsMag0=0  IrMag0=0  IsAngle0=0  IrAngle0=0
  Ground3 : spsGroundLib/Ground  LConnTagsString=a
  "Grounding Transformer " : spsGroundingTransformerLib/Grounding Transformer   UNITS=pu  NominalPower="[100e6   60]"  NominalVoltage=25e3  ZeroSequenceImpedance_pu=[0.025 0.75]  MagnetizationBranch_pu=[500 500]  ZeroSequenceImpedance_SI=[0.052083 589.05]  MagnetizationBranch_SI=[1041.7 3.927e+005]  Measurements=None
  A : PMIOPort  Side=Left
  B : PMIOPort  Port=2  Side=Left
  C : PMIOPort  Port=3  Side=Left
  connections:
  "3.3ohms "/RConn1 -- Ground3/LConn1
  120 kV / 25 kV 47 MVA/LConn1 -- 120kV 2500MVA/RConn1
  120 kV / 25 kV 47 MVA/LConn2 -- 120kV 2500MVA/RConn2
  120 kV / 25 kV 47 MVA/LConn3 -- 120kV 2500MVA/RConn3
  120 kV / 25 kV 47 MVA/RConn1 -- "Grounding Transformer "/LConn1 -- 14-km Feeder/RConn1 -- 30-MW 2-Mvar Load/LConn1
  120 kV / 25 kV 47 MVA/RConn2 -- "Grounding Transformer "/LConn2 -- 14-km Feeder/RConn2 -- 30-MW 2-Mvar Load/LConn2
  120 kV / 25 kV 47 MVA/RConn3 -- "Grounding Transformer "/LConn3 -- 14-km Feeder/RConn3 -- 30-MW 2-Mvar Load/LConn3
  5-km Feeder/RConn1 -- 14-km Feeder/LConn1 -- 2-MW Load/LConn1
  5-km Feeder/RConn2 -- 14-km Feeder/LConn2 -- 2-MW Load/LConn2
  5-km Feeder/RConn3 -- 14-km Feeder/LConn3 -- 2-MW Load/LConn3
  A/RConn1 -- 5-km Feeder/LConn1
  B/RConn1 -- 5-km Feeder/LConn2
  C/RConn1 -- 5-km Feeder/LConn3
  "Grounding Transformer "/RConn1 -- "3.3ohms "/LConn1

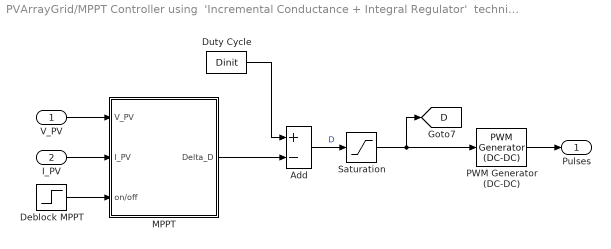
== system PVArrayGrid/MPPT Controller using  'Incremental Conductance + Integral Regulator'  technique  ==
  V_PV : Inport
  I_PV : Inport  Port=2
  Add : Sum  Inputs=+-
  Deblock MPPT : Step  Time=0.4  SampleTime=0
  Duty Cycle : Constant  Value=Dinit
  MPPT : Subsystem
  PWM Generator (DC-DC) : spsPWMGeneratorDCDCLib/PWM Generator (DC-DC)  Fsw=fc  Ts=Ts_Power
  Saturation : Saturate  UpperLimit=1  LowerLimit=0
  Pulses : Outport  VectorParamsAs1DForOutWhenUnconnected=off
  tag scope: D=global
  wires:
  V_PV/1 -> MPPT/1(V_PV)
  I_PV/1 -> MPPT/2(I_PV)
  PWM Generator (DC-DC)/1 -> Pulses/1
  Deblock MPPT/1 -> MPPT/3(on/off)
  Saturation/1 -> PWM Generator (DC-DC)/1, [D]
  Add/1 -> Saturation/1  "D"
  MPPT/1(Delta_D) -> Add/2
  Duty Cycle/1 -> Add/1

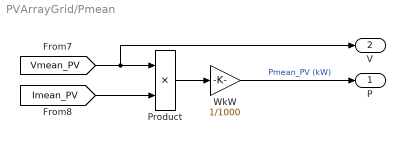
== system PVArrayGrid/Pmean ==
  Product : Product  RndMeth=Zero
  WkW : Gain  Gain=1/1000
  P : Outport  VectorParamsAs1DForOutWhenUnconnected=off
  V : Outport  Port=2  VectorParamsAs1DForOutWhenUnconnected=off
  wires:
  [Vmean_PV] -> Product/1, V/1
  Product/1 -> WkW/1
  [Imean_PV] -> Product/2
  WkW/1 -> P/1  "Pmean_PV (kW)"

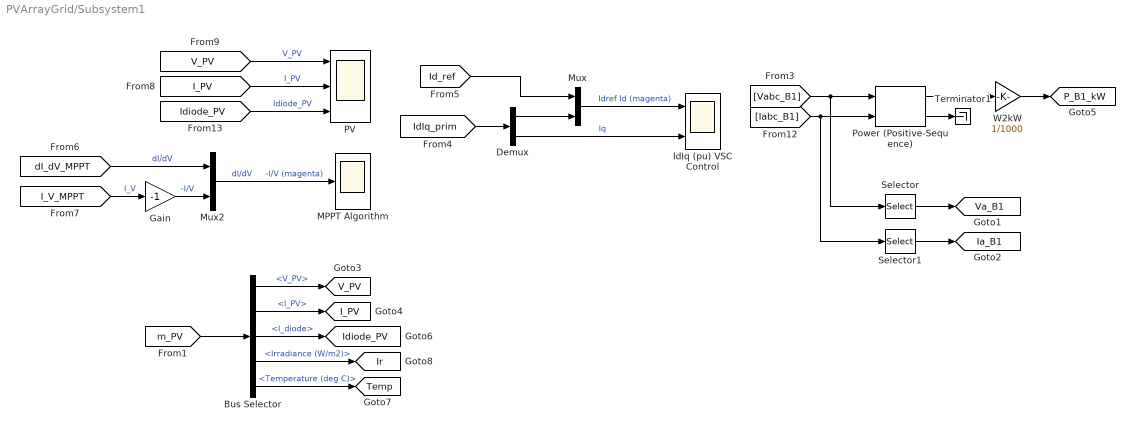
== system PVArrayGrid/Subsystem1 ==
  Bus Selector : BusSelector  OutputSignals=V_PV,I_PV,I_diode,Irradiance (W/m2),Temperature (deg C)
  Demux : Demux  Outputs=2
  Gain : Gain  Gain=-1
  IdIq (pu) VSC Control : Scope  NumInputPorts=2
  MPPT Algorithm : Scope
  Mux : Mux  Inputs=2
  Mux2 : Mux  Inputs=2
  PV : Scope  NumInputPorts=3
  Power (Positive-Sequence) : spsPowerPositiveSequenceLib/Power (Positive-Sequence)  Freq=60  Vinit=[0, 0]  Iinit=[0, 0]  Ts=Ts_Control
  Selector : Selector  InputPortWidth=3  IndexOptions=Index vector (dialog)  Indices=[1]  OutputSizes=1
  Selector1 : Selector  InputPortWidth=3  IndexOptions=Index vector (dialog)  Indices=[1]  OutputSizes=1
  Terminator1 : Terminator
  W2kW : Gain  Gain=1/1000
  tag scope: I_PV=global, Ia_B1=global, Idiode_PV=global, Ir=global, P_B1_kW=global, Temp=global, V_PV=global, Va_B1=global
  wires:
  [Vabc_B1] -> Power (Positive-Sequence)/1, Selector/1
  [Iabc_B1] -> Power (Positive-Sequence)/2, Selector1/1
  Power (Positive-Sequence)/1 -> W2kW/1
  [I_V_MPPT] -> Gain/1  "I_V"
  [IdIq_prim] -> Demux/1
  [Id_ref] -> Mux/1
  Demux/1 -> Mux/2
  Mux/1 -> IdIq (pu) VSC Control/1  "Idref Id (magenta)"
  Demux/2 -> IdIq (pu) VSC Control/2  "Iq"
  Selector/1 -> [Va_B1]
  Selector1/1 -> [Ia_B1]
  [V_PV] -> PV/1  "V_PV"
  [I_PV] -> PV/2  "I_PV"
  [Idiode_PV] -> PV/3  "Idiode_PV"
  [dI_dV_MPPT] -> Mux2/1  "dI/dV"
  Gain/1 -> Mux2/2  "-I/V"
  Mux2/1 -> MPPT Algorithm/1  "dI/dV     -I/V (magenta)"
  W2kW/1 -> [P_B1_kW]
  [m_PV] -> Bus Selector/1
  Bus Selector/1 -> [V_PV]  "<V_PV>"
  Bus Selector/2 -> [I_PV]  "<I_PV>"
  Bus Selector/4 -> [Ir]  "<Irradiance (W/m2)>"
  Bus Selector/3 -> [Idiode_PV]  "<I_diode>"
  Bus Selector/5 -> [Temp]  "<Temperature (deg C)>"
  Power (Positive-Sequence)/2 -> Terminator1/1

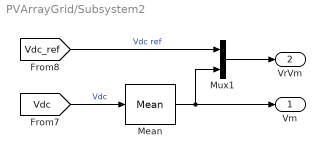
== system PVArrayGrid/Subsystem2 ==
  Mean : spsMeanLib/Mean  Freq=60  Vinit=0  Ts=Ts_Control
  Mux1 : Mux  Inputs=2
  Vm : Outport  VectorParamsAs1DForOutWhenUnconnected=off
  VrVm : Outport  Port=2  VectorParamsAs1DForOutWhenUnconnected=off
  wires:
  [Vdc_ref] -> Mux1/1  "Vdc ref"
  [Vdc] -> Mean/1  "Vdc"
  Mux1/1 -> VrVm/1
  Mean/1 -> Mux1/2, Vm/1

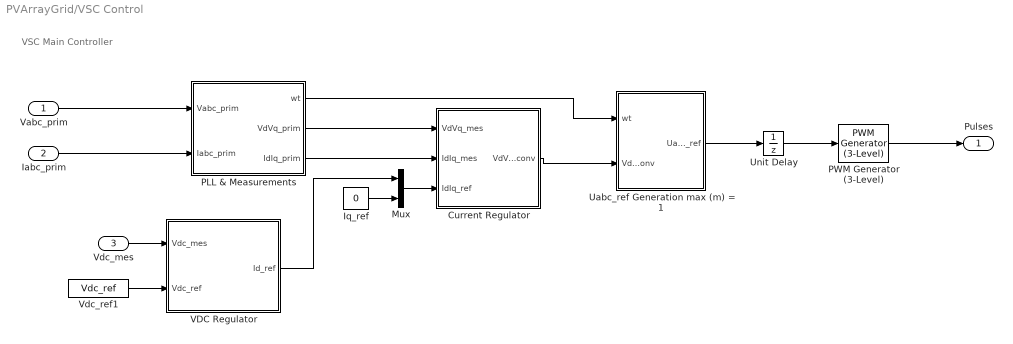
== system PVArrayGrid/VSC Control ==
  note: VSC Main Controller
  Vabc_prim : Inport  PortDimensions=3
  Iabc_prim : Inport  Port=2  PortDimensions=3
  Vdc_mes : Inport  Port=3  PortDimensions=1
  Current Regulator : Subsystem
  Iq_ref : Constant  Value=0
  Mux : Mux  Inputs=2
  PLL & Measurements : Subsystem
  PWM Generator (3-Level) : spsPWMGenerator3LevelLib/PWM Generator (3-Level)  ModulatorType=Three-phase bridge (12 pulses)  ModulatorMode=Unsynchronized  nF=27  Fc=33*60  ModulatingSignals=off  m=0.8  Freq=60  Phase=0  Ts=Ts_Power
  Uabc_ref Generation max (m) = 1 : Subsystem
  Unit Delay : UnitDelay  SampleTime=Ts_Control  HasFrameUpgradeWarning=on
  VDC Regulator : Subsystem
  Vdc_ref1 : Constant  Value=Vdc_ref
  Pulses : Outport  VectorParamsAs1DForOutWhenUnconnected=off
  wires:
  VDC Regulator/1(Id_ref) -> Mux/1
  PLL & Measurements/1(wt) -> Uabc_ref Generation max (m) = 1/1(wt)
  Current Regulator/1(VdVq_conv) -> Uabc_ref Generation max (m) = 1/2(VdVq_conv)
  Iq_ref/1 -> Mux/2
  Mux/1 -> Current Regulator/3(IdIq_ref)
  PLL & Measurements/3(IdIq_prim) -> Current Regulator/2(IdIq_mes)
  PLL & Measurements/2(VdVq_prim) -> Current Regulator/1(VdVq_mes)
  Vdc_mes/1 -> VDC Regulator/1(Vdc_mes)
  Vabc_prim/1 -> PLL & Measurements/1(Vabc_prim)
  Iabc_prim/1 -> PLL & Measurements/2(Iabc_prim)
  Unit Delay/1 -> PWM Generator (3-Level)/1
  PWM Generator (3-Level)/1 -> Pulses/1
  Uabc_ref Generation max (m) = 1/1(Uabc_ref) -> Unit Delay/1
  Vdc_ref1/1 -> VDC Regulator/2(Vdc_ref)

== system PVArrayGrid/info ==

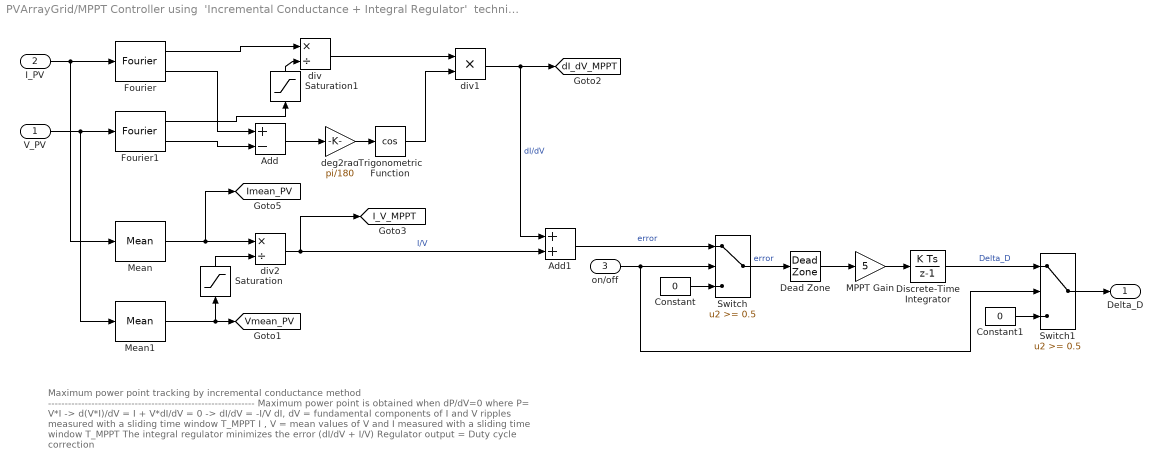
== system PVArrayGrid/MPPT Controller using  'Incremental Conductance + Integral Regulator'  technique /MPPT ==
  note: Maximum power point tracking by incremental conductance method
      | --------------------------------------------------------------
      | Maximum power point is obtained when dP/dV=0  where P= V*I
      | -> d(V*I)/dV = I + V*dI/dV = 0
      | -> dI/dV = -I/V
      |
      | dI, dV  = fundamental components of I and V ripples measured with a sliding time window T_MPPT
      | I , V   = mean values of V and I measured with a sliding time window T_MPPT
      |
      | The integral regulator minimizes the error (dI/dV + I/V)
      | Regulator output = Duty cycle correction
  V_PV : Inport
  I_PV : Inport  Port=2
  on/off : Inport  Port=3
  Add : Sum  Inputs=+-
  Add1 : Sum
  Constant : Constant  Value=0
  Constant1 : Constant  Value=0
  Dead Zone : DeadZone  LowerValue=-0.05  UpperValue=0.05
  Discrete-Time Integrator : DiscreteIntegrator  SampleTime=Ts_Control  LimitOutput=on  UpperSaturationLimit=1  LowerSaturationLimit=-1  ICPrevOutput=DiscIntNeverNeededParam  ICPrevScaledInput=DiscIntNeverNeededParam
  Fourier : spsFourierLib/Fourier  Freq=1/T_MPPT  n=1  InInit=[0, 0]  Ts=Ts_Control
  Fourier1 : spsFourierLib/Fourier  Freq=1/T_MPPT  n=1  InInit=[0, 0]  Ts=Ts_Control
  MPPT Gain : Gain  Gain=5
  Mean : spsMeanLib/Mean  Freq=1/T_MPPT  Vinit=0  Ts=Ts_Control
  Mean1 : spsMeanLib/Mean  Freq=1/T_MPPT  Vinit=0  Ts=Ts_Control
  Saturation : Saturate  UpperLimit=inf  LowerLimit=eps
  Saturation1 : Saturate  UpperLimit=inf  LowerLimit=eps
  Switch : Switch  Threshold=0.5  SaturateOnIntegerOverflow=off  InputSameDT=off
  Switch1 : Switch  Threshold=0.5  SaturateOnIntegerOverflow=off  InputSameDT=off
  Trigonometric Function : Trigonometry  Operator=cos
  deg2rad : Gain  Gain=pi/180
  div : Product  Inputs=*/  RndMeth=Zero
  div1 : Product  Inputs=**  RndMeth=Zero
  div2 : Product  Inputs=*/  RndMeth=Zero
  Delta_D : Outport  VectorParamsAs1DForOutWhenUnconnected=off
  tag scope: I_V_MPPT=global, Imean_PV=global, Vmean_PV=global, dI_dV_MPPT=global
  wires:
  Dead Zone/1 -> MPPT Gain/1
  Switch/1 -> Dead Zone/1  "error"
  Saturation1/1 -> div/2
  Saturation/1 -> div2/2
  Switch1/1 -> Delta_D/1
  on/off/1 -> Switch/2, Switch1/2
  Constant1/1 -> Switch1/3
  Discrete-Time Integrator/1 -> Switch1/1  "Delta_D"
  Constant/1 -> Switch/3
  MPPT Gain/1 -> Discrete-Time Integrator/1
  Add1/1 -> Switch/1  "error"
  div2/1 -> Add1/2, [I_V_MPPT]  "I/V"
  Mean1/1 -> Saturation/1, [Vmean_PV]
  Mean/1 -> div2/1, [Imean_PV]
  div1/1 -> Add1/1, [dI_dV_MPPT]  "dI/dV"
  Trigonometric Function/1 -> div1/2
  div/1 -> div1/1
  deg2rad/1 -> Trigonometric Function/1
  Add/1 -> deg2rad/1
  Fourier1/1 -> Saturation1/1
  Fourier1/2 -> Add/2
  Fourier/2 -> Add/1
  V_PV/1 -> Mean1/1, Fourier1/1
  I_PV/1 -> Mean/1, Fourier/1
  Fourier/1 -> div/1
